simulink model "m301825"  (Simulink 6.5)
settings: Solver=ode3  SolverMode=SingleTasking  StartTime=0.0  StopTime=2000  FixedStep=0.01  RelTol=1e-5  AbsTol=1e-6
CloseFcn:
  | rtwprivate ssgencode ModelCloseRequest ssdemo
settings Model: Creator=nikita  LastModifiedBy=mshakeri  ExtModeTrigMode=oneshot  ExtModeArmWhenConnect=off  ExtModeAutoUpdateStatusClock=off
settings DataIOCC: LimitDataPoints=off  SaveOutput=off  SaveTime=off  SignalLoggingName=sigsOut
settings OptimizationCC: InlineParams=on  InlineInvariantSignals=on  EnforceIntegerDowncast=off  StateBitsets=on  DataBitsets=on  UseTempVars=on  ZeroExternalMemoryAtStartup=off  ZeroInternalMemoryAtStartup=off  InitFltsAndDblsToZero=off  LifeSpan=1
settings DebuggingCC: SignalResolutionControl=UseLocalSettings  SolverPrmCheckMsg=none  MultiTaskDSMMsg=warning  MultiTaskCondExecSysMsg=none  IntegerOverflowMsg=none  StrictBusMsg=ErrorLevel1
settings RTWCC: SystemTargetFile=ert.tlc  TLCOptions=-p0  TemplateMakefile=ert_default_tmf  GenerateReport=on  RetainRTWFile=on  ProcessScript=ert_make_rtw_hook  IncludeHyperlinkInReport=on  LaunchReport=on
settings CodeAppCC: IgnoreCustomStorageClasses=off  PrefixModelToSubsysFcnNames=off
settings ERTTargetCC: TargetFcnLib=ansi_tfl_tmw.mat  GenFloatMathFcnCalls=ANSI_C  GenerateSampleERTMain=on  IncludeMdlTerminateFcn=off  IncludeERTFirstTime=on  GenerateErtSFunction=on  ERTSrcFileBannerTemplate=example_banner.tlc  ERTHdrFileBannerTemplate=example_banner.tlc  ERTDataSrcFileTemplate=example_banner.tlc  ERTDataHdrFileTemplate=example_banner.tlc  ERTCustomFileTemplate=example_file_process.tlc  InitialValueSource=Model

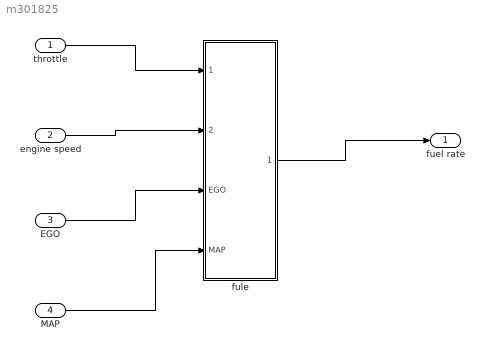
== system m301825 ==
  throttle : Inport  SampleTime=.01
  engine speed : Inport  Port=2  SampleTime=.01
  EGO : Inport  Port=3  SampleTime=.01
  MAP : Inport  Port=4  SampleTime=.01
  fule : Subsystem
  fuel rate : Outport  InitialOutput=0
  wires:
  fule/1(fuel rate) -> fuel rate/1
  throttle/1 -> fule/1(throttle)
  engine speed/1 -> fule/2(engine speed)
  EGO/1 -> fule/3(EGO)
  MAP/1 -> fule/4(MAP)

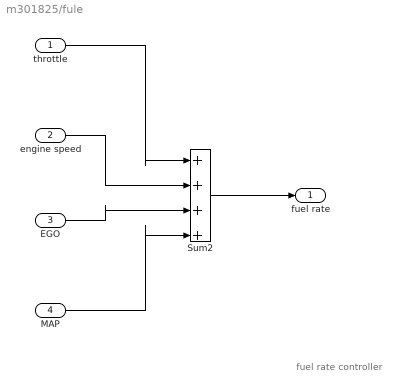
== system m301825/fule ==
  note: fuel rate controller
  throttle : Inport  SampleTime=.01
  engine speed : Inport  Port=2  SampleTime=.01
  EGO : Inport  Port=3  SampleTime=.01
  MAP : Inport  Port=4  SampleTime=.01
  Sum2 : Sum  Inputs=++++  SaturateOnIntegerOverflow=on  InputSameDT=on
  fuel rate : Outport  InitialOutput=0
  wires:
  throttle/1 -> Sum2/1
  engine speed/1 -> Sum2/2
  EGO/1 -> Sum2/3
  MAP/1 -> Sum2/4
  Sum2/1 -> fuel rate/1
